simulink model "BatteryPackAttempt1"  (R2024a)
settings: Solver=VariableStepAuto  StartTime=0.0  StopTime=10.0  RelTol=1e-3
undefined symbols (not defined in the file): Ion, Lithium
libraries: spsBatteryLib x32, sps_lib x1
settings Model: Creator=RGUKT  LastModifiedBy=RGUKT

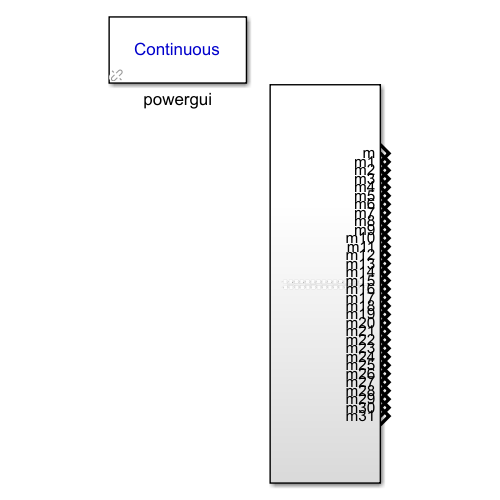
[thumbnail: Simulink's stored preview of the top-level diagram]
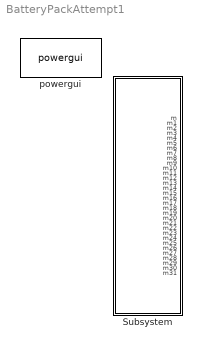
== system BatteryPackAttempt1 ==
  Subsystem : Subsystem
  powergui : sps_lib/powergui  Priority=1  SimulationMode=Continuous  SampleTime=50e-6  frequency=60  Iterations=50  frequencyindice=0  Pbase=100e6  ErrMax=1e-4  UnitsV=kV  UnitsW=MW  buscounter=0  FunctionMessages=off  echomessages=off  EnableUseOfTLC=off  CurrentSourceSwitches=off  DisableSnubberDevices=off  DisableRonSwitches=off  DisableVfSwitches=off  DisplayEquations=off  AutomaticDiscreteSolvers=off  SolverType=Tustin/Backward Euler (TBE)  Interpol=off  ExternalGateDelay=off  methode=off  Ts=100  x0status=blocks  SPID=on  SwTol=0  HookPort=off  NonlinearTolerance=1e-4  nMaxIteration=100  ContinueOnMaxIteration=off  RestoreLinks=warning  ResistiveCurrentMeasurement=off  Frange=[0:2:500]  Ylog=off  Xlog=on  ShowGrid=off  save=off  variable=ZData  structure=0  ZoomFFT=off  StartTime=0.0  cycles=1  DisplayStyle=1  fundamental=60  FreqAxis=off  MaxFrequency=1000  frequencyindicesteady=1  RmsSteady=1  display=off

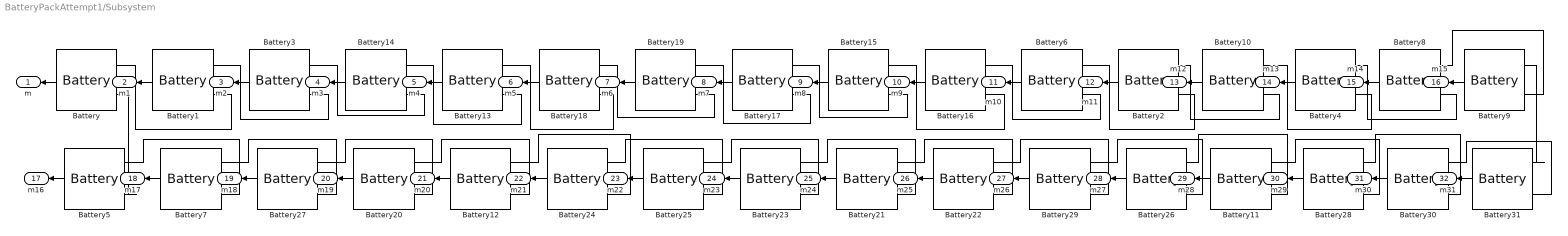
== system BatteryPackAttempt1/Subsystem ==
  Battery{,1..31} (32 alike) : spsBatteryLib/Battery  BatType=Lithium-Ion  ShowTempParam=off  ThermalPreset=no  ShowAgeParam=off  NomV=7.2  NomQ=5.4  SOC=100  Batt_Tr=30  PresetModel=on  MaxQ=5.4  MinV=5.4  FullV=8.3807  Dis_rate=2.3478  R=0.013333  Normal_OP=4.8835  expZone="[7.7788      0.2653]"  current=[6.5 13 32.5]  Units=Time  Tci=20  NomT=20  T2=-30  MaxQ2=4.8  FullV2=7.1  Normal_OP2=5.655  expZone2="[6.58           1]"  Rca=0.6  ti=2000  Dp=0  Neq0=0  Tsim=1e6  Ta1=25  Qeol=5.4*0.9  Reol=0.013333*1.2  Char_age=[2.3478, 3]  Dis_age=[2.3478, 10]  N1=1500  N2=10500  N3=1000  N4=1400  Ta2=45  N5=950
  m : Outport
  m1 : Outport  Port=2
  m2 : Outport  Port=3
  m3 : Outport  Port=4
  m4 : Outport  Port=5
  m5 : Outport  Port=6
  m6 : Outport  Port=7
  m7 : Outport  Port=8
  m8 : Outport  Port=9
  m9 : Outport  Port=10
  m10 : Outport  Port=11
  m11 : Outport  Port=12
  m12 : Outport  Port=13
  m13 : Outport  Port=14
  m14 : Outport  Port=15
  m15 : Outport  Port=16
  m16 : Outport  Port=17
  m17 : Outport  Port=18
  m18 : Outport  Port=19
  m19 : Outport  Port=20
  m20 : Outport  Port=21
  m21 : Outport  Port=22
  m22 : Outport  Port=23
  m23 : Outport  Port=24
  m24 : Outport  Port=25
  m25 : Outport  Port=26
  m26 : Outport  Port=27
  m27 : Outport  Port=28
  m28 : Outport  Port=29
  m29 : Outport  Port=30
  m30 : Outport  Port=31
  m31 : Outport  Port=32
  wires:
  Battery8/1 -> m14/1
  Battery19/1 -> m6/1
  Battery30/1 -> m30/1
  Battery7/1 -> m17/1
  Battery27/1 -> m18/1
  Battery22/1 -> m25/1
  Battery21/1 -> m24/1
  Battery3/1 -> m2/1
  Battery20/1 -> m19/1
  Battery5/1 -> m16/1
  Battery25/1 -> m22/1
  Battery18/1 -> m5/1
  Battery15/1 -> m8/1
  Battery26/1 -> m27/1
  Battery1/1 -> m1/1
  Battery29/1 -> m26/1
  Battery2/1 -> m11/1
  Battery24/1 -> m21/1
  Battery13/1 -> m4/1
  Battery/1 -> m/1
  Battery4/1 -> m13/1
  Battery14/1 -> m3/1
  Battery6/1 -> m10/1
  Battery9/1 -> m15/1
  Battery11/1 -> m28/1
  Battery10/1 -> m12/1
  Battery12/1 -> m20/1
  Battery16/1 -> m9/1
  Battery23/1 -> m23/1
  Battery28/1 -> m29/1
  Battery31/1 -> m31/1
  Battery17/1 -> m7/1
  connections:
  Battery30/LConn1 -- Battery31/LConn2
  Battery6/LConn1 -- Battery2/LConn2
  Battery2/LConn1 -- Battery10/LConn2
  Battery/LConn1 -- Battery1/LConn2
  Battery21/LConn1 -- Battery22/LConn2
  Battery31/LConn1 -- Battery9/LConn1
  Battery15/LConn1 -- Battery16/LConn2
  Battery14/LConn1 -- Battery13/LConn2
  Battery30/LConn2 -- Battery28/LConn1
  Battery5/LConn2 -- Battery/LConn2
  Battery11/LConn1 -- Battery28/LConn2
  Battery22/LConn1 -- Battery29/LConn2
  Battery3/LConn1 -- Battery14/LConn2
  Battery18/LConn1 -- Battery19/LConn2
  Battery1/LConn1 -- Battery3/LConn2
  Battery4/LConn1 -- Battery8/LConn2
  Battery7/LConn1 -- Battery27/LConn2
  Battery19/LConn1 -- Battery17/LConn2
  Battery5/LConn1 -- Battery7/LConn2
  Battery26/LConn1 -- Battery11/LConn2
  Battery23/LConn1 -- Battery21/LConn2
  Battery25/LConn1 -- Battery23/LConn2
  Battery24/LConn1 -- Battery25/LConn2
  Battery16/LConn1 -- Battery6/LConn2
  Battery10/LConn1 -- Battery4/LConn2
  Battery8/LConn1 -- Battery9/LConn2
  Battery20/LConn1 -- Battery12/LConn2
  Battery13/LConn1 -- Battery18/LConn2
  Battery27/LConn1 -- Battery20/LConn2
  Battery29/LConn1 -- Battery26/LConn2
  Battery17/LConn1 -- Battery15/LConn2
  Battery12/LConn1 -- Battery24/LConn2
